simulink model "dynamic_modeling"  (R2021a)
settings: Solver=VariableStepAuto  StartTime=0.0  StopTime=30  RelTol=1e-3
libraries: robotmobilelib x1, simulink x1
settings Model: Creator=THANH DAT  LastModifiedBy=THANH DAT

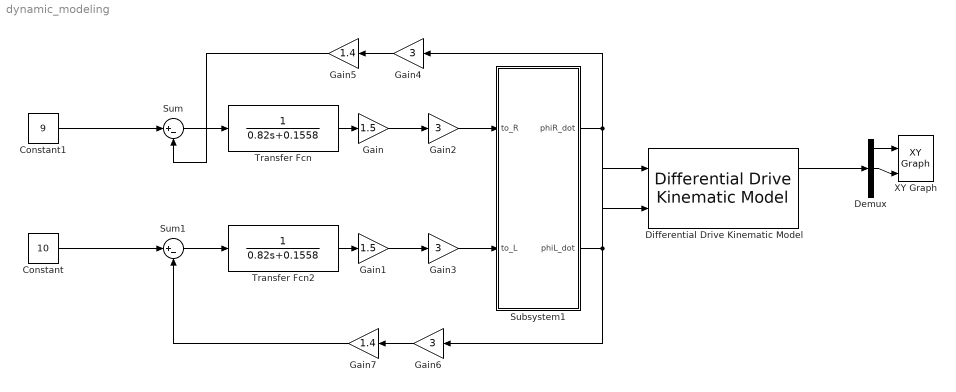
== system dynamic_modeling ==
  Constant : Constant  Value=10
  Constant1 : Constant  Value=9
  Demux : Demux  Outputs=3
  Differential Drive Kinematic Model : robotmobilelib/Differential Drive Kinematic Model  VehicleInputs=Wheel Speeds  WheelRadius=0.07  WheelSpeedRange=[-inf inf]  TrackWidth=0.2  InitialState=[0; 0; 0]  SimulateUsing=Interpreted execution
      settings: SourceProductBaseCode=RO
  Gain : Gain  Gain=1.5
  Gain1 : Gain  Gain=1.5
  Gain{2..4,6} (4 alike) : Gain  Gain=3
  Gain5 : Gain  Gain=1.4
  Gain7 : Gain  Gain=1.4
  Subsystem1 : Subsystem
  Sum : Sum  Inputs=|+-
  Sum1 : Sum  Inputs=|+-
  Transfer Fcn : TransferFcn  Denominator=[ 0.82 0.1558]
  Transfer Fcn2 : TransferFcn  Denominator=[ 0.82 0.1558]
  XY Graph : simulink/Sinks/XY Graph  xmin=-10  xmax=10  ymin=-20  ymax=20  st=-1
  wires:
  Sum/1 -> Transfer Fcn/1
  Sum1/1 -> Transfer Fcn2/1
  Transfer Fcn/1 -> Gain/1
  Transfer Fcn2/1 -> Gain1/1
  Gain/1 -> Gain2/1
  Gain1/1 -> Gain3/1
  Gain2/1 -> Subsystem1/1("to_R ")
  Gain3/1 -> Subsystem1/2(to_L)
  Subsystem1/1(phiR_dot) -> Gain4/1, Differential Drive Kinematic Model/2
  Gain4/1 -> Gain5/1
  Gain5/1 -> Sum/2
  Gain6/1 -> Gain7/1
  Subsystem1/2(phiL_dot) -> Gain6/1, Differential Drive Kinematic Model/1
  Gain7/1 -> Sum1/2
  Constant1/1 -> Sum/1
  Constant/1 -> Sum1/1
  Differential Drive Kinematic Model/1 -> Demux/1
  Demux/1 -> XY Graph/1
  Demux/2 -> XY Graph/2

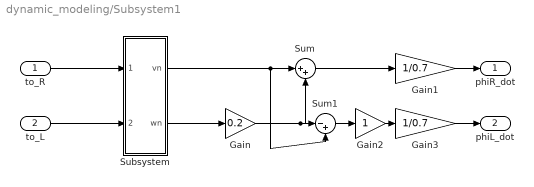
== system dynamic_modeling/Subsystem1 ==
  "to_R " : Inport
  to_L : Inport  Port=2
  Gain : Gain  Gain=0.2
  Gain1 : Gain  Gain=1/0.7
  Gain2 : Gain
  Gain3 : Gain  Gain=1/0.7
  Subsystem : Subsystem
  Sum : Sum  Inputs=|++
  Sum1 : Sum  Inputs=|-+
  phiR_dot : Outport
  phiL_dot : Outport  Port=2
  wires:
  Subsystem/1(vn) -> Sum/1, Sum1/2
  Subsystem/2(wn) -> Gain/1
  Sum1/1 -> Gain2/1
  Gain/1 -> Sum/2, Sum1/1
  Gain1/1 -> phiR_dot/1
  "to_R "/1 -> Subsystem/1("to_R ")
  Gain2/1 -> Gain3/1
  Gain3/1 -> phiL_dot/1
  Sum/1 -> Gain1/1
  to_L/1 -> Subsystem/2(to_L)

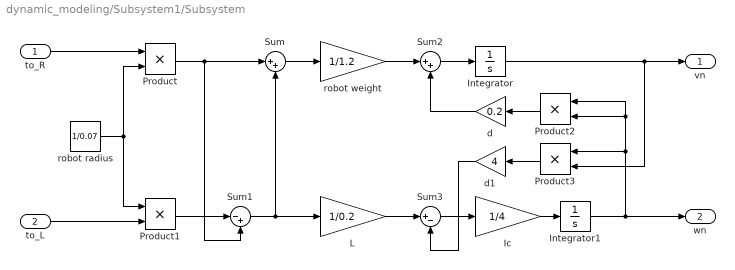
== system dynamic_modeling/Subsystem1/Subsystem ==
  "to_R " : Inport
  to_L : Inport  Port=2
  Ic : Gain  Gain=1/4
  Integrator : Integrator
  Integrator1 : Integrator
  L : Gain  Gain=1/0.2
  Product{,1..3} (4 alike) : Product
  Sum : Sum  Inputs=|++
  Sum1 : Sum  Inputs=|-+
  Sum2 : Sum  Inputs=|++
  Sum3 : Sum  Inputs=|+-
  d : Gain  Gain=0.2
  d1 : Gain  Gain=4
  "robot radius " : Constant  Value=1/0.07
  robot weight : Gain  Gain=1/1.2
  vn : Outport
  wn : Outport  Port=2
  wires:
  Product2/1 -> d/1
  Sum/1 -> robot weight/1
  Sum3/1 -> Ic/1
  d/1 -> Sum2/2
  to_L/1 -> Product1/2
  Integrator1/1 -> wn/1, Product3/1, Product2/2, Product2/1
  L/1 -> Sum3/1
  "robot radius "/1 -> Product/2, Product1/1
  Sum1/1 -> L/1, Sum/2
  Product1/1 -> Sum1/1
  robot weight/1 -> Sum2/1
  Integrator/1 -> vn/1, Product3/2
  "to_R "/1 -> Product/1
  Product/1 -> Sum/1, Sum1/2
  Ic/1 -> Integrator1/1
  Sum2/1 -> Integrator/1
  d1/1 -> Sum3/2
  Product3/1 -> d1/1
